simulink model "V2X_Core_Simulink_model"  (R2023b)
settings: Solver=VariableStepAuto  StartTime=0.0  StopTime=210  MaxStep=1e-2  RelTol=1e-3  AbsTol=1e-3
values from neighbouring files (symbols this model uses):
  b = 1.6    [a2024_v2x_matlab_6veh.m]
  mEgo = 1500    [a2024_v2x_matlab_6veh.m]
  Mode = 1    [a2024_v2x_matlab_6veh.m]    (also in v2x_matlab.m; v2x_matlabV2.m; v2x_matlab_6veh.m; v2x_matlab_R.m)
  pilot = (randi(s,[0 1],pilotsPerSym,1)-0.5)*2    [v2x_matlab.m]
  RxPower = [waypoints, ss']    [v2x_matlab.m]    (also in v2x_matlab_6veh.m)
  sampleTime = 0.1    [a2024_v2x_matlab_6veh.m]    (also in v2x_matlab.m; v2x_matlabV2.m; v2x_matlab_6veh.m; v2x_matlab_R.m)
  t_gap = 1.4    [a2024_v2x_matlab_6veh.m]
  waypoints = [egoWP(:,2) egoWP(:,1), zeroforwp]    [a2024_v2x_matlab_6veh.m]    (also in misc.m = data.data.ActorSpecifications(1,1).Waypoints(:,[1,2]); v2x_matlab.m = data.data.ActorSpecifications(1,1).Waypoints(:,[1,2]); v2x_matlabV2.m = [5 -1.6 0; v2x_matlab_R.m = [5 -1.6 0)
  ZeroActors = struct(     'ActorID',0,     'Position', [1000 1000 1000],      'Velocity', [0 0 0],      'Roll', 0,      'Pitch', 0,      'Yaw', 0,      'AngularVelocity', [0 0 0])    [v2x_matlabV2.m]    (also in v2x_matlab_R.m)
undefined symbols (not defined in the file or in its folder): driving, PredictionHorizon, Ts
libraries: commofdm x21, simulink x16, commdigbbndam3 x14, simulink_extras x12, commcnvcod2 x11, commdigbbndpm3 x9, commblkintrlv2 x4, drivingscenarioandsensors x3, mpcadaslib x2, vehdynlibdriver x1, autolibshared x1, commchan3 x1
(part 2 of 4)

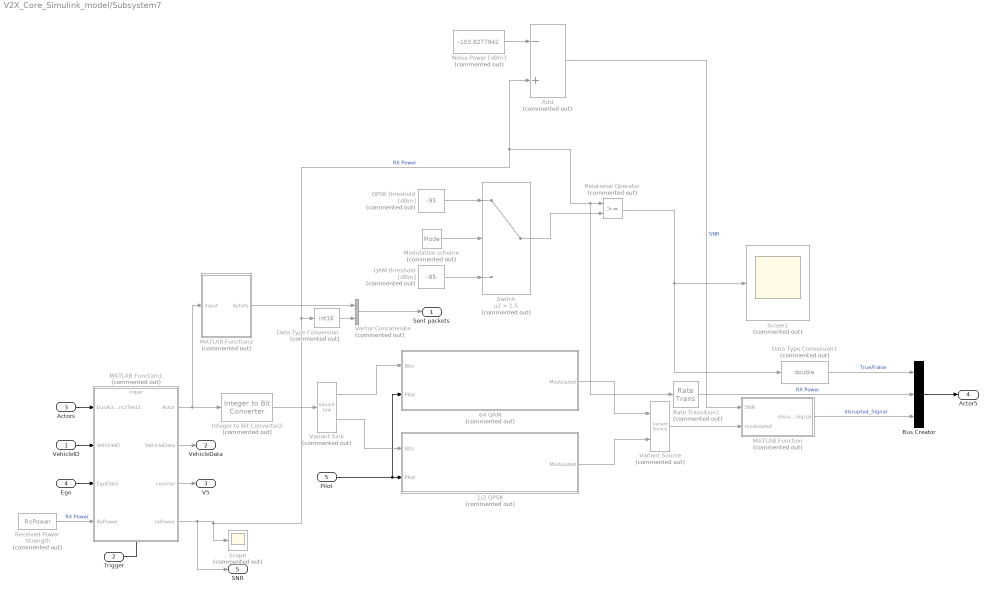
== system V2X_Core_Simulink_model/Subsystem7 ==
  VehicleID : Inport
  Trigger : Inport  Port=2
  Actors : Inport  Port=3
  Ego : Inport  Port=4
  Pilot : Inport  Port=5
  1/2 QPSK : Subsystem  Commented=on  TreatAsAtomicUnit=on
  64 QAM : Subsystem  Commented=on  TreatAsAtomicUnit=on
  Add : Sum  Commented=on  Inputs=-+
  Bus Creator : BusCreator  Inputs=3
  Data Type Conversion : DataTypeConversion  Commented=on  OutDataTypeStr=int16  SaturateOnIntegerOverflow=off  RndMeth=Floor
  Data Type Conversion1 : DataTypeConversion  Commented=on  OutDataTypeStr=double  SaturateOnIntegerOverflow=off  RndMeth=Floor
  Integer to Bit Converter2 : simulink/Logic and Bit Operations/Integer to Bit Converter  Commented=on  nbits=16  signedInputValues=Signed  bitOrder=MSB first  outDtype=boolean
  MATLAB Function : MATLAB Function  Commented=on  TreatAsAtomicUnit=on
  MATLAB Function1 : MATLAB Function  Commented=on  TreatAsAtomicUnit=on
  MATLAB Function2 : MATLAB Function  Commented=on  TreatAsAtomicUnit=on  SystemSampleTime=0.01
  Modulation scheme : Constant  Commented=on  Value=Mode
  Noise Power [dBm] : Constant  Commented=on  Value=-103.8277942
  QAM threshold [dBm] : Constant  Commented=on  Value=-85
  QPSK threshold [dBm] : Constant  Commented=on  Value=-95
  Rate Transition1 : RateTransition  Commented=on  OutPortSampleTime=sampleTime/10
  Received Power Strength : Constant  Commented=on  Value=RxPower
  Relational Operator : RelationalOperator  Commented=on  OutDataTypeStr=boolean  RndMeth=Simplest  InputSameDT=off
  Scope : Scope  Commented=on
  Scope1 : Scope  Commented=on
  Switch : Switch  Commented=on  Criteria=u2 > Threshold  Threshold=1.5  SaturateOnIntegerOverflow=off  InputSameDT=off
  Variant Sink : VariantSink  Commented=on
  Variant Source : VariantSource  Commented=on
  Vector Concatenate : Concatenate  Commented=on
  Sent packets : Outport
  VehicleData : Outport  Port=2
  V5 : Outport  Port=3
  Actor5 : Outport  Port=4
  SNR : Outport  Port=5
  wires:
  MATLAB Function1/1(Actor) -> MATLAB Function2/1(input), Integer to Bit Converter2/1
  Ego/1 -> MATLAB Function1/3(EgoData)
  Actors/1 -> MATLAB Function1/1(busActors3Test1)
  VehicleID/1 -> MATLAB Function1/2(VehicleID)
  MATLAB Function1/2(VehicleData) -> VehicleData/1
  MATLAB Function1/3(counter) -> V5/1
  Trigger/1 -> MATLAB Function1/Trigger
  Integer to Bit Converter2/1 -> Variant Sink/1
  Pilot/1 -> 64 QAM/2(Pilot), 1/2 QPSK/2(Pilot)
  64 QAM/1(Modulated) -> Variant Source/1
  1/2 QPSK/1(Modulated) -> Variant Source/2
  Variant Source/1 -> MATLAB Function/2(modulated)
  Variant Sink/1 -> 64 QAM/1(Bits)
  Variant Sink/2 -> 1/2 QPSK/1(Bits)
  Noise Power [dBm]/1 -> Add/1
  QPSK threshold [dBm]/1 -> Switch/1
  QAM threshold [dBm]/1 -> Switch/3
  Modulation scheme/1 -> Switch/2
  Add/1 -> MATLAB Function/1(SNR)  "SNR"
  Switch/1 -> Relational Operator/2
  Relational Operator/1 -> Data Type Conversion1/1, Scope1/1
  MATLAB Function1/4(rxPower) -> Data Type Conversion/1, Rate Transition1/1, Relational Operator/1, Add/2, Scope/1, SNR/1  "RX Power"
  Received Power Strength/1 -> MATLAB Function1/4(RxPower)  "RX Power"
  Bus Creator/1 -> Actor5/1
  MATLAB Function2/1(Actors) -> Vector Concatenate/1
  Vector Concatenate/1 -> Sent packets/1
  MATLAB Function/1(disrupted_Signal) -> Bus Creator/3  "disrupted_Signal"
  Data Type Conversion/1 -> Vector Concatenate/2
  Data Type Conversion1/1 -> Bus Creator/1  "True/False"
  Rate Transition1/1 -> Bus Creator/2  "RX Power"

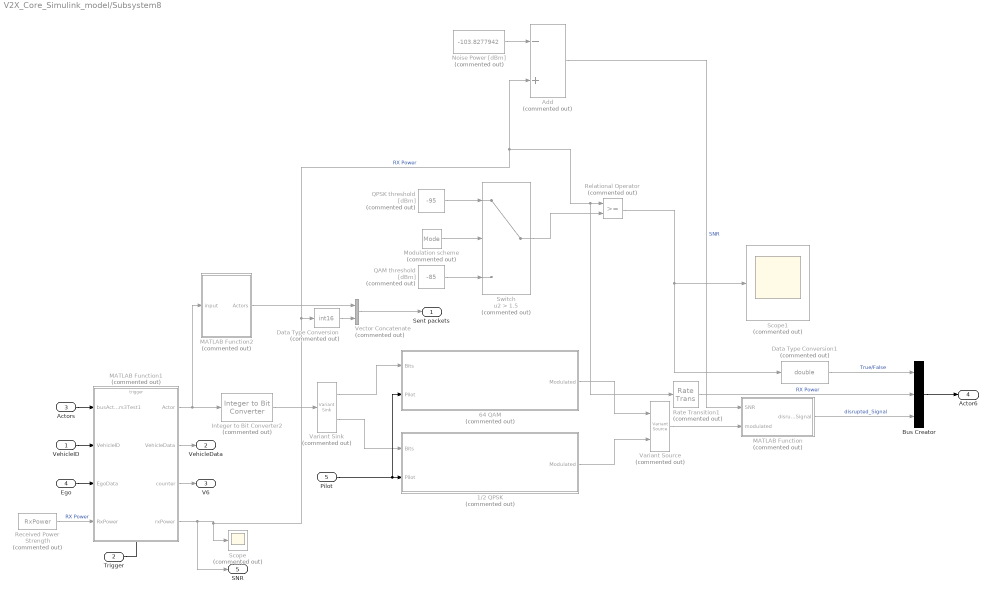
== system V2X_Core_Simulink_model/Subsystem8 ==
  VehicleID : Inport
  Trigger : Inport  Port=2
  Actors : Inport  Port=3
  Ego : Inport  Port=4
  Pilot : Inport  Port=5
  1/2 QPSK : Subsystem  Commented=on  TreatAsAtomicUnit=on
  64 QAM : Subsystem  Commented=on  TreatAsAtomicUnit=on
  Add : Sum  Commented=on  Inputs=-+
  Bus Creator : BusCreator  Inputs=3
  Data Type Conversion : DataTypeConversion  Commented=on  OutDataTypeStr=int16  SaturateOnIntegerOverflow=off  RndMeth=Floor
  Data Type Conversion1 : DataTypeConversion  Commented=on  OutDataTypeStr=double  SaturateOnIntegerOverflow=off  RndMeth=Floor
  Integer to Bit Converter2 : simulink/Logic and Bit Operations/Integer to Bit Converter  Commented=on  nbits=16  signedInputValues=Signed  bitOrder=MSB first  outDtype=boolean
  MATLAB Function : MATLAB Function  Commented=on  TreatAsAtomicUnit=on
  MATLAB Function1 : MATLAB Function  Commented=on  TreatAsAtomicUnit=on
  MATLAB Function2 : MATLAB Function  Commented=on  TreatAsAtomicUnit=on  SystemSampleTime=0.01
  Modulation scheme : Constant  Commented=on  Value=Mode
  Noise Power [dBm] : Constant  Commented=on  Value=-103.8277942
  QAM threshold [dBm] : Constant  Commented=on  Value=-85
  QPSK threshold [dBm] : Constant  Commented=on  Value=-95
  Rate Transition1 : RateTransition  Commented=on  OutPortSampleTime=sampleTime/10
  Received Power Strength : Constant  Commented=on  Value=RxPower
  Relational Operator : RelationalOperator  Commented=on  OutDataTypeStr=boolean  RndMeth=Simplest  InputSameDT=off
  Scope : Scope  Commented=on
  Scope1 : Scope  Commented=on
  Switch : Switch  Commented=on  Criteria=u2 > Threshold  Threshold=1.5  SaturateOnIntegerOverflow=off  InputSameDT=off
  Variant Sink : VariantSink  Commented=on
  Variant Source : VariantSource  Commented=on
  Vector Concatenate : Concatenate  Commented=on
  Sent packets : Outport
  VehicleData : Outport  Port=2
  V6 : Outport  Port=3
  Actor6 : Outport  Port=4
  SNR : Outport  Port=5
  wires:
  Rate Transition1/1 -> Bus Creator/2  "RX Power"
  Data Type Conversion1/1 -> Bus Creator/1  "True/False"
  Data Type Conversion/1 -> Vector Concatenate/2
  MATLAB Function/1(disrupted_Signal) -> Bus Creator/3  "disrupted_Signal"
  Vector Concatenate/1 -> Sent packets/1
  MATLAB Function2/1(Actors) -> Vector Concatenate/1
  Bus Creator/1 -> Actor6/1
  Received Power Strength/1 -> MATLAB Function1/4(RxPower)  "RX Power"
  MATLAB Function1/4(rxPower) -> SNR/1, Scope/1, Add/2, Relational Operator/1, Rate Transition1/1, Data Type Conversion/1  "RX Power"
  Relational Operator/1 -> Scope1/1, Data Type Conversion1/1
  Switch/1 -> Relational Operator/2
  Add/1 -> MATLAB Function/1(SNR)  "SNR"
  Modulation scheme/1 -> Switch/2
  QAM threshold [dBm]/1 -> Switch/3
  QPSK threshold [dBm]/1 -> Switch/1
  Noise Power [dBm]/1 -> Add/1
  Variant Sink/2 -> 1/2 QPSK/1(Bits)
  Variant Sink/1 -> 64 QAM/1(Bits)
  Variant Source/1 -> MATLAB Function/2(modulated)
  1/2 QPSK/1(Modulated) -> Variant Source/2
  64 QAM/1(Modulated) -> Variant Source/1
  Pilot/1 -> 1/2 QPSK/2(Pilot), 64 QAM/2(Pilot)
  Integer to Bit Converter2/1 -> Variant Sink/1
  Trigger/1 -> MATLAB Function1/Trigger
  MATLAB Function1/3(counter) -> V6/1
  MATLAB Function1/2(VehicleData) -> VehicleData/1
  VehicleID/1 -> MATLAB Function1/2(VehicleID)
  Actors/1 -> MATLAB Function1/1(busActors3Test1)
  Ego/1 -> MATLAB Function1/3(EgoData)
  MATLAB Function1/1(Actor) -> Integer to Bit Converter2/1, MATLAB Function2/1(input)

== system V2X_Core_Simulink_model/Vehicle 2 ==
  trigger : Inport
  VehicleID : Inport  Port=2
  Pilot : Inport  Port=3
  busActors3Test1 : Inport  Port=4
  Constant2 : Constant  Value=[zeros(19,1)']  SampleTime=-1
  Entity Multicast1 : EntityMulticast  InputPortMessageModes=m
  Integer to Bit Converter1 : simulink/Logic and Bit Operations/Integer to Bit Converter  nbits=16  signedInputValues=Signed  bitOrder=MSB first  outDtype=boolean
  MATLAB Function1 : MATLAB Function  TreatAsAtomicUnit=on
  OFDM Modulator1 : commofdm/OFDM Modulator  StatePerturbationForJacobian=1.0e-05  FFTLength=64  NumGuardBandCarriers=[0;0]  InsertDCNull=on  PilotInputPort=on  PilotCarrierIndices=[12; 26; 40; 54]  CyclicPrefixLength=32  Windowing=off  WindowLength=16  OversamplingFactor=3  NumSymbols=1  NumTransmitAntennas=1  SimulateUsing=Interpreted execution
  Rectangular QAM Modulator Baseband1 : commdigbbndam3/Rectangular QAM Modulator Baseband  M=2^6  InType=Bit  Enc=Binary  Mapping=[0:15]  PowType=Average Power  MinDist=2  AvgPow=P_Signal  PeakPow=1  Ph=0  outDtype=double  outWordLen=16  outUDDataType=sfix(16)  outFracLenMode=Best precision  outFracLen=15  outDataTypeStr=double  outLastDataTypeStr=double
      settings: LibrarySourceBlock=|
      | commhdldigbbndam/Rectangular QAM
      | Modulator
      | Baseband
  Send1 : Send  OutputPortMessageModes=m
  Vector Concatenate1 : Concatenate
  wires:
  busActors3Test1/1 -> MATLAB Function1/1(busActors3Test1)
  Rectangular QAM Modulator Baseband1/1 -> Vector Concatenate1/1
  Constant2/1 -> Vector Concatenate1/2
  Send1/1 -> Entity Multicast1/1
  Integer to Bit Converter1/1 -> Rectangular QAM Modulator Baseband1/1
  Vector Concatenate1/1 -> OFDM Modulator1/1  "After QAM Mod"
  OFDM Modulator1/1 -> Send1/1  "OFDM modulated"
  MATLAB Function1/1(intVector) -> Integer to Bit Converter1/1
  trigger/1 -> MATLAB Function1/Trigger
  VehicleID/1 -> MATLAB Function1/2(VehicleID)
  Pilot/1 -> OFDM Modulator1/2

== system V2X_Core_Simulink_model/Vehicle 3 ==
  trigger : Inport
  busActors3Test1 : Inport  Port=2
  Pilot : Inport  Port=3
  VehicleID : Inport  Port=4
  Constant3 : Constant  Value=[zeros(19,1)']  SampleTime=-1
  Entity Multicast2 : EntityMulticast  InputPortMessageModes=m
  Integer to Bit Converter3 : simulink/Logic and Bit Operations/Integer to Bit Converter  nbits=16  signedInputValues=Signed  bitOrder=MSB first  outDtype=boolean
  MATLAB Function2 : MATLAB Function  TreatAsAtomicUnit=on
  OFDM Modulator2 : commofdm/OFDM Modulator  StatePerturbationForJacobian=1.0e-05  FFTLength=64  NumGuardBandCarriers=[0;0]  InsertDCNull=on  PilotInputPort=on  PilotCarrierIndices=[12; 26; 40; 54]  CyclicPrefixLength=32  Windowing=off  WindowLength=16  OversamplingFactor=3  NumSymbols=1  NumTransmitAntennas=1  SimulateUsing=Interpreted execution
  Rectangular QAM Modulator Baseband3 : commdigbbndam3/Rectangular QAM Modulator Baseband  M=2^6  InType=Bit  Enc=Binary  Mapping=[0:15]  PowType=Average Power  MinDist=2  AvgPow=P_Signal  PeakPow=1  Ph=0  outDtype=double  outWordLen=16  outUDDataType=sfix(16)  outFracLenMode=Best precision  outFracLen=15  outDataTypeStr=double  outLastDataTypeStr=double
      settings: LibrarySourceBlock=|
      | commhdldigbbndam/Rectangular QAM
      | Modulator
      | Baseband
  Send2 : Send  OutputPortMessageModes=m
  Vector Concatenate2 : Concatenate
  wires:
  MATLAB Function2/1(intVector) -> Integer to Bit Converter3/1
  OFDM Modulator2/1 -> Send2/1  "OFDM modulated"
  busActors3Test1/1 -> MATLAB Function2/1(busActors3Test1)
  Vector Concatenate2/1 -> OFDM Modulator2/1  "After QAM Mod"
  Send2/1 -> Entity Multicast2/1
  Integer to Bit Converter3/1 -> Rectangular QAM Modulator Baseband3/1
  Rectangular QAM Modulator Baseband3/1 -> Vector Concatenate2/1
  Pilot/1 -> OFDM Modulator2/2
  Constant3/1 -> Vector Concatenate2/2
  VehicleID/1 -> MATLAB Function2/2(VehicleID)
  trigger/1 -> MATLAB Function2/Trigger

== system V2X_Core_Simulink_model/ACC/Lane Keeping Assist ==
  Longitudinal velocity of ego : Inport
  Enable : Inport  Port=2
  Lane Assist Offset : Inport  Port=3
  lane boundaries Bus : Inport  Port=4
  Driver Steer : Inport  Port=5
  Abs : Abs  SaturateOnIntegerOverflow=off
  Estimate lane center : Subsystem
  Lane Keeping Assist System : mpcadaslib/Lane Keeping Assist System  ModelType=Use vehicle parameters  VehicleMass=mEgo  VehicleYawInertia=2875  LengthToFront=a  LengthToRear=b  FrontTireStiffness=Cy_f  RearTireStiffness=Cy_r  EgoModelMatrixA=[-4.4021 ,-12.4603;1.3913,-5.1868]  EgoModelMatrixB=[24.1270;15.8609]  EgoModelMatrixC=[1,0;0,1]  InitialLongVel=16  TransportLag=0  MinSteering=-0.5  umin_ext=off  MaxSteering=0.5  umax_ext=off  Ts=0.1  PredictionHorizon=5  ControllerBehavior=0.100  suboptimal=off  maxiter=10  datatypeopt=double  optmode=off  trackmode=off
      link override Longitudinal velocity must be positive: stopWhenAssertionFail=on
      settings: LibrarySourceBlock=mpclib/Automated Driving/Lane Keeping Assist System
  Pack to Custom Sensor Data Format : Subsystem
  Subsystem : Subsystem
  Subsystem2 : Subsystem
  Vision Detection Generator : drivingscenarioandsensors/Vision Detection Generator  SensorIndex=1  DetectorOutput=Lanes only  UpdateInterval=0.1  LaneUpdateInterval=0.1  SensorLocation=[ 1.9, 0 ]  Height=1.1  Yaw=0  Pitch=1  Roll=0  BusNameSource=Auto  BusName=BusObjectDetections  BusName2Source=Auto  BusName2=BusLaneDetections  MaxNumDetectionsSource=Property  MaxNumDetections=50  MaxNumLanesSource=Property  MaxNumLanes=30  DetectionCoordinates=Ego Cartesian  SimulateUsing=Interpreted execution  MaxRange=10  BoundingBoxAccuracy=5  ProcessNoiseIntensity=5  MaxSpeed=100  MaxAllowedOcclusion=0.5  MinObjectImageSize=[ 15, 15 ]  DetectionProbability=0.9  FalsePositivesPerImage=0.1  MinLaneImageSize=[ 20, 3 ]  LaneBoundaryAccuracy=3  HasNoise=on  InitialSeedSource=Repeatable  InitialSeed=0  UsedSeed=driving.internal.SimulinkUtilities.seedManager(gcb)  ActorProfilesSource=From Scenario Reader block  ActorProfilesParameters=driving.internal.ActorProfilesParameters  ActorProfilesExpression=struct( 'ClassID', 0, 'Length', 4.7, 'Width', 1.8, 'Height', 1.4, 'OriginOffset', [ -1.35, 0, 0 ] )  Intrinsics=driving.internal.cameraIntrinsics('FocalLength',[1, 1 ])
  Status : Outport
  SteeringAngle in rad : Outport  Port=2
  wires:
  Subsystem/1(Departure Detected) -> Subsystem2/2(Set)
  Estimate lane center/2(Lateral Offset) -> Lane Keeping Assist System/3
  Enable/1 -> Subsystem2/1(Enable)
  Pack to Custom Sensor Data Format/1(lanes) -> Subsystem/2(Lane Sensor data), Estimate lane center/2(Lane Boundaries)
  Estimate lane center/1(Previewed Curvature) -> Lane Keeping Assist System/1
  Estimate lane center/3(Heading Angle) -> Lane Keeping Assist System/4
  lane boundaries Bus/1 -> Vision Detection Generator/1
  Vision Detection Generator/1 -> Pack to Custom Sensor Data Format/1(lane Detections)
  Lane Assist Offset/1 -> Subsystem/1(Lane Assist Offset)
  Driver Steer/1 -> Subsystem2/4(Driver Steer)
  Subsystem2/1(Status) -> Status/1
  Longitudinal velocity of ego/1 -> Abs/1, Estimate lane center/1(Longitudinal velocity of ego)
  Abs/1 -> Lane Keeping Assist System/2
  Subsystem2/2(SteeringAngle in rad) -> SteeringAngle in rad/1
  Lane Keeping Assist System/1 -> Subsystem2/3(Assisted Steer)  "Assisted Steer"

== system V2X_Core_Simulink_model/Calculate PDR/PDR V1 ==
  Sent packet : Inport
  Received packets : Inport  Port=2
  Vehicle ID : Inport  Port=3
  Add : Sum  Commented=on  Inputs=-+
  Bus Selector3 : BusSelector  Commented=on  OutputSignals=ActorID,Position,Velocity,Roll,Pitch,Yaw,AngularVelocity
  Constant : Constant  Commented=on
  Data Type Conversion1 : DataTypeConversion  Commented=on  OutDataTypeStr=double  SaturateOnIntegerOverflow=off  RndMeth=Floor
  MATLAB Function : MATLAB Function  TreatAsAtomicUnit=on
  MATLAB Function1 : MATLAB Function  TreatAsAtomicUnit=on
  MATLAB Function2 : MATLAB Function  TreatAsAtomicUnit=on
  MATLAB Function6 : MATLAB Function  Commented=on  TreatAsAtomicUnit=on
  Matrix Concatenate : Concatenate  Mode=Multidimensional array  ConcatenateDimension=2
  Round : Rounding  Commented=on  Operator=round
  Selector : Selector  Commented=through  IndexOptions=Starting index (dialog)  Indices=3  OutputSizes=13
  Transpose : Math  Commented=on  Operator=transpose
  Vector Concatenate1 : Concatenate  Commented=on  NumInputs=7
  PDR1 : Outport
  Vectors output : Outport  Port=2
  wires:
  MATLAB Function2/1(y) -> Selector/1
  Received packets/1 -> MATLAB Function2/2(u)
  MATLAB Function1/1(y) -> Matrix Concatenate/1, MATLAB Function/1(Tx)
  MATLAB Function/1(PDR) -> PDR1/1
  Matrix Concatenate/1 -> Vectors output/1
  Selector/1 -> MATLAB Function/2(Rx), Matrix Concatenate/2
  Vehicle ID/1 -> MATLAB Function1/2(Vehicle_ID), MATLAB Function2/1(Vehicle_ID)
  ? -> MATLAB Function6/2(vehicleID)
  Bus Selector3/6 -> Vector Concatenate1/6  "<Yaw>"
  Bus Selector3/4 -> Vector Concatenate1/4  "<Roll>"
  Constant/1 -> Add/1
  Bus Selector3/7 -> Vector Concatenate1/7  "<AngularVelocity>"
  Vector Concatenate1/1 -> Transpose/1
  Add/1 -> Vector Concatenate1/1
  MATLAB Function6/1(y) -> Bus Selector3/1
  Bus Selector3/3 -> Vector Concatenate1/3  "<Velocity>"
  Bus Selector3/2 -> Vector Concatenate1/2  "<Position>"
  ? -> MATLAB Function6/1(u)
  Bus Selector3/5 -> Vector Concatenate1/5  "<Pitch>"
  Bus Selector3/1 -> Add/2  "<ActorID>"
  Transpose/1 -> Round/1
  Round/1 -> Data Type Conversion1/1
  Sent packet/1 -> MATLAB Function1/1(u)

== system V2X_Core_Simulink_model/Calculate PDR/PDR V2 ==
  Sent packet : Inport
  Received packets : Inport  Port=2
  Vehicle ID : Inport  Port=3
  Add : Sum  Commented=on  Inputs=-+
  Bus Selector3 : BusSelector  Commented=on  OutputSignals=ActorID,Position,Velocity,Roll,Pitch,Yaw,AngularVelocity
  Constant : Constant  Commented=on
  Data Type Conversion1 : DataTypeConversion  Commented=on  OutDataTypeStr=double  SaturateOnIntegerOverflow=off  RndMeth=Floor
  MATLAB Function : MATLAB Function  TreatAsAtomicUnit=on
  MATLAB Function1 : MATLAB Function  TreatAsAtomicUnit=on
  MATLAB Function2 : MATLAB Function  TreatAsAtomicUnit=on
  MATLAB Function6 : MATLAB Function  Commented=on  TreatAsAtomicUnit=on
  Matrix Concatenate : Concatenate  Mode=Multidimensional array  ConcatenateDimension=2
  Round : Rounding  Commented=on  Operator=round
  Selector : Selector  Commented=through  IndexOptions=Starting index (dialog)  Indices=3  OutputSizes=13
  Transpose : Math  Commented=on  Operator=transpose
  Vector Concatenate1 : Concatenate  Commented=on  NumInputs=7
  PDR1 : Outport
  Vectors output : Outport  Port=2
  wires:
  Sent packet/1 -> MATLAB Function1/1(u)
  Round/1 -> Data Type Conversion1/1
  Transpose/1 -> Round/1
  Bus Selector3/1 -> Add/2  "<ActorID>"
  Bus Selector3/5 -> Vector Concatenate1/5  "<Pitch>"
  ? -> MATLAB Function6/1(u)
  Bus Selector3/2 -> Vector Concatenate1/2  "<Position>"
  Bus Selector3/3 -> Vector Concatenate1/3  "<Velocity>"
  MATLAB Function6/1(y) -> Bus Selector3/1
  Add/1 -> Vector Concatenate1/1
  Vector Concatenate1/1 -> Transpose/1
  Bus Selector3/7 -> Vector Concatenate1/7  "<AngularVelocity>"
  Constant/1 -> Add/1
  Bus Selector3/4 -> Vector Concatenate1/4  "<Roll>"
  Bus Selector3/6 -> Vector Concatenate1/6  "<Yaw>"
  ? -> MATLAB Function6/2(vehicleID)
  Vehicle ID/1 -> MATLAB Function2/1(Vehicle_ID), MATLAB Function1/2(Vehicle_ID)
  Selector/1 -> Matrix Concatenate/2, MATLAB Function/2(Rx)
  Matrix Concatenate/1 -> Vectors output/1
  MATLAB Function/1(PDR) -> PDR1/1
  MATLAB Function1/1(y) -> MATLAB Function/1(Tx), Matrix Concatenate/1
  Received packets/1 -> MATLAB Function2/2(u)
  MATLAB Function2/1(y) -> Selector/1

== system V2X_Core_Simulink_model/Calculate PDR/PDR V3 ==
  Sent packet : Inport
  Received packets : Inport  Port=2
  Vehicle ID : Inport  Port=3
  Add : Sum  Commented=on  Inputs=-+
  Bus Selector3 : BusSelector  Commented=on  OutputSignals=ActorID,Position,Velocity,Roll,Pitch,Yaw,AngularVelocity
  Constant : Constant  Commented=on
  Data Type Conversion1 : DataTypeConversion  Commented=on  OutDataTypeStr=double  SaturateOnIntegerOverflow=off  RndMeth=Floor
  MATLAB Function : MATLAB Function  TreatAsAtomicUnit=on
  MATLAB Function1 : MATLAB Function  TreatAsAtomicUnit=on
  MATLAB Function2 : MATLAB Function  TreatAsAtomicUnit=on
  MATLAB Function6 : MATLAB Function  Commented=on  TreatAsAtomicUnit=on
  Matrix Concatenate : Concatenate  Mode=Multidimensional array  ConcatenateDimension=2
  Round : Rounding  Commented=on  Operator=round
  Selector : Selector  Commented=through  IndexOptions=Starting index (dialog)  Indices=3  OutputSizes=13
  Transpose : Math  Commented=on  Operator=transpose
  Vector Concatenate1 : Concatenate  Commented=on  NumInputs=7
  PDR1 : Outport
  Vectors output : Outport  Port=2
  wires:
  MATLAB Function2/1(y) -> Selector/1
  Received packets/1 -> MATLAB Function2/2(u)
  MATLAB Function1/1(y) -> Matrix Concatenate/1, MATLAB Function/1(Tx)
  MATLAB Function/1(PDR) -> PDR1/1
  Matrix Concatenate/1 -> Vectors output/1
  Selector/1 -> MATLAB Function/2(Rx), Matrix Concatenate/2
  Vehicle ID/1 -> MATLAB Function1/2(Vehicle_ID), MATLAB Function2/1(Vehicle_ID)
  ? -> MATLAB Function6/2(vehicleID)
  Bus Selector3/6 -> Vector Concatenate1/6  "<Yaw>"
  Bus Selector3/4 -> Vector Concatenate1/4  "<Roll>"
  Constant/1 -> Add/1
  Bus Selector3/7 -> Vector Concatenate1/7  "<AngularVelocity>"
  Vector Concatenate1/1 -> Transpose/1
  Add/1 -> Vector Concatenate1/1
  MATLAB Function6/1(y) -> Bus Selector3/1
  Bus Selector3/3 -> Vector Concatenate1/3  "<Velocity>"
  Bus Selector3/2 -> Vector Concatenate1/2  "<Position>"
  ? -> MATLAB Function6/1(u)
  Bus Selector3/5 -> Vector Concatenate1/5  "<Pitch>"
  Bus Selector3/1 -> Add/2  "<ActorID>"
  Transpose/1 -> Round/1
  Round/1 -> Data Type Conversion1/1
  Sent packet/1 -> MATLAB Function1/1(u)

== system V2X_Core_Simulink_model/Calculate PDR/PDR V4 ==
  Sent packet : Inport
  Received packets : Inport  Port=2
  Vehicle ID : Inport  Port=3
  Add : Sum  Commented=on  Inputs=-+
  Bus Selector3 : BusSelector  Commented=on  OutputSignals=ActorID,Position,Velocity,Roll,Pitch,Yaw,AngularVelocity
  Constant : Constant  Commented=on
  Data Type Conversion1 : DataTypeConversion  Commented=on  OutDataTypeStr=double  SaturateOnIntegerOverflow=off  RndMeth=Floor
  MATLAB Function : MATLAB Function  TreatAsAtomicUnit=on
  MATLAB Function1 : MATLAB Function  TreatAsAtomicUnit=on
  MATLAB Function2 : MATLAB Function  TreatAsAtomicUnit=on
  MATLAB Function6 : MATLAB Function  Commented=on  TreatAsAtomicUnit=on
  Matrix Concatenate : Concatenate  Mode=Multidimensional array  ConcatenateDimension=2
  Round : Rounding  Commented=on  Operator=round
  Selector : Selector  Commented=through  IndexOptions=Starting index (dialog)  Indices=3  OutputSizes=13
  Transpose : Math  Commented=on  Operator=transpose
  Vector Concatenate1 : Concatenate  Commented=on  NumInputs=7
  PDR1 : Outport
  Vectors output : Outport  Port=2
  wires:
  Sent packet/1 -> MATLAB Function1/1(u)
  Round/1 -> Data Type Conversion1/1
  Transpose/1 -> Round/1
  Bus Selector3/1 -> Add/2  "<ActorID>"
  Bus Selector3/5 -> Vector Concatenate1/5  "<Pitch>"
  ? -> MATLAB Function6/1(u)
  Bus Selector3/2 -> Vector Concatenate1/2  "<Position>"
  Bus Selector3/3 -> Vector Concatenate1/3  "<Velocity>"
  MATLAB Function6/1(y) -> Bus Selector3/1
  Add/1 -> Vector Concatenate1/1
  Vector Concatenate1/1 -> Transpose/1
  Bus Selector3/7 -> Vector Concatenate1/7  "<AngularVelocity>"
  Constant/1 -> Add/1
  Bus Selector3/4 -> Vector Concatenate1/4  "<Roll>"
  Bus Selector3/6 -> Vector Concatenate1/6  "<Yaw>"
  ? -> MATLAB Function6/2(vehicleID)
  Vehicle ID/1 -> MATLAB Function2/1(Vehicle_ID), MATLAB Function1/2(Vehicle_ID)
  Selector/1 -> Matrix Concatenate/2, MATLAB Function/2(Rx)
  Matrix Concatenate/1 -> Vectors output/1
  MATLAB Function/1(PDR) -> PDR1/1
  MATLAB Function1/1(y) -> MATLAB Function/1(Tx), Matrix Concatenate/1
  Received packets/1 -> MATLAB Function2/2(u)
  MATLAB Function2/1(y) -> Selector/1

== system V2X_Core_Simulink_model/Calculate PDR/PDR V5 ==
  Sent packet : Inport
  Received packets : Inport  Port=2
  Vehicle ID : Inport  Port=3
  Add : Sum  Commented=on  Inputs=-+
  Bus Selector3 : BusSelector  Commented=on  OutputSignals=ActorID,Position,Velocity,Roll,Pitch,Yaw,AngularVelocity
  Constant : Constant  Commented=on
  Data Type Conversion1 : DataTypeConversion  Commented=on  OutDataTypeStr=double  SaturateOnIntegerOverflow=off  RndMeth=Floor
  MATLAB Function : MATLAB Function  TreatAsAtomicUnit=on
  MATLAB Function1 : MATLAB Function  TreatAsAtomicUnit=on
  MATLAB Function2 : MATLAB Function  TreatAsAtomicUnit=on
  MATLAB Function6 : MATLAB Function  Commented=on  TreatAsAtomicUnit=on
  Matrix Concatenate : Concatenate  Mode=Multidimensional array  ConcatenateDimension=2
  Round : Rounding  Commented=on  Operator=round
  Selector : Selector  Commented=through  IndexOptions=Starting index (dialog)  Indices=3  OutputSizes=13
  Transpose : Math  Commented=on  Operator=transpose
  Vector Concatenate1 : Concatenate  Commented=on  NumInputs=7
  PDR1 : Outport
  Vectors output : Outport  Port=2
  wires:
  MATLAB Function2/1(y) -> Selector/1
  Received packets/1 -> MATLAB Function2/2(u)
  MATLAB Function1/1(y) -> Matrix Concatenate/1, MATLAB Function/1(Tx)
  MATLAB Function/1(PDR) -> PDR1/1
  Matrix Concatenate/1 -> Vectors output/1
  Selector/1 -> MATLAB Function/2(Rx), Matrix Concatenate/2
  Vehicle ID/1 -> MATLAB Function1/2(Vehicle_ID), MATLAB Function2/1(Vehicle_ID)
  ? -> MATLAB Function6/2(vehicleID)
  Bus Selector3/6 -> Vector Concatenate1/6  "<Yaw>"
  Bus Selector3/4 -> Vector Concatenate1/4  "<Roll>"
  Constant/1 -> Add/1
  Bus Selector3/7 -> Vector Concatenate1/7  "<AngularVelocity>"
  Vector Concatenate1/1 -> Transpose/1
  Add/1 -> Vector Concatenate1/1
  MATLAB Function6/1(y) -> Bus Selector3/1
  Bus Selector3/3 -> Vector Concatenate1/3  "<Velocity>"
  Bus Selector3/2 -> Vector Concatenate1/2  "<Position>"
  ? -> MATLAB Function6/1(u)
  Bus Selector3/5 -> Vector Concatenate1/5  "<Pitch>"
  Bus Selector3/1 -> Add/2  "<ActorID>"
  Transpose/1 -> Round/1
  Round/1 -> Data Type Conversion1/1
  Sent packet/1 -> MATLAB Function1/1(u)

== system V2X_Core_Simulink_model/Calculate PDR/PDR V6 ==
  Sent packet : Inport
  Received packets : Inport  Port=2
  Vehicle ID : Inport  Port=3
  Add : Sum  Commented=on  Inputs=-+
  Bus Selector3 : BusSelector  Commented=on  OutputSignals=ActorID,Position,Velocity,Roll,Pitch,Yaw,AngularVelocity
  Constant : Constant  Commented=on
  Data Type Conversion1 : DataTypeConversion  Commented=on  OutDataTypeStr=double  SaturateOnIntegerOverflow=off  RndMeth=Floor
  MATLAB Function : MATLAB Function  TreatAsAtomicUnit=on
  MATLAB Function1 : MATLAB Function  TreatAsAtomicUnit=on
  MATLAB Function2 : MATLAB Function  TreatAsAtomicUnit=on
  MATLAB Function6 : MATLAB Function  Commented=on  TreatAsAtomicUnit=on
  Matrix Concatenate : Concatenate  Mode=Multidimensional array  ConcatenateDimension=2
  Round : Rounding  Commented=on  Operator=round
  Selector : Selector  Commented=through  IndexOptions=Starting index (dialog)  Indices=3  OutputSizes=13
  Transpose : Math  Commented=on  Operator=transpose
  Vector Concatenate1 : Concatenate  Commented=on  NumInputs=7
  PDR1 : Outport
  Vectors output : Outport  Port=2
  wires:
  Sent packet/1 -> MATLAB Function1/1(u)
  Round/1 -> Data Type Conversion1/1
  Transpose/1 -> Round/1
  Bus Selector3/1 -> Add/2  "<ActorID>"
  Bus Selector3/5 -> Vector Concatenate1/5  "<Pitch>"
  ? -> MATLAB Function6/1(u)
  Bus Selector3/2 -> Vector Concatenate1/2  "<Position>"
  Bus Selector3/3 -> Vector Concatenate1/3  "<Velocity>"
  MATLAB Function6/1(y) -> Bus Selector3/1
  Add/1 -> Vector Concatenate1/1
  Vector Concatenate1/1 -> Transpose/1
  Bus Selector3/7 -> Vector Concatenate1/7  "<AngularVelocity>"
  Constant/1 -> Add/1
  Bus Selector3/4 -> Vector Concatenate1/4  "<Roll>"
  Bus Selector3/6 -> Vector Concatenate1/6  "<Yaw>"
  ? -> MATLAB Function6/2(vehicleID)
  Vehicle ID/1 -> MATLAB Function2/1(Vehicle_ID), MATLAB Function1/2(Vehicle_ID)
  Selector/1 -> Matrix Concatenate/2, MATLAB Function/2(Rx)
  Matrix Concatenate/1 -> Vectors output/1
  MATLAB Function/1(PDR) -> PDR1/1
  MATLAB Function1/1(y) -> MATLAB Function/1(Tx), Matrix Concatenate/1
  Received packets/1 -> MATLAB Function2/2(u)
  MATLAB Function2/1(y) -> Selector/1

== system V2X_Core_Simulink_model/Queue/Switch Case Action Subsystem ==
  Actor1 : Inport
  Action Port : ActionPort  ActionPortLabel=case [ 0 ]:
  Out1 : Outport
  wires:
  Actor1/1 -> Out1/1

== system V2X_Core_Simulink_model/Queue/Switch Case Action Subsystem1 ==
  Actor1 : Inport
  Action Port : ActionPort  ActionPortLabel=case [ 1 ]:
  Out1 : Outport
  wires:
  Actor1/1 -> Out1/1

== system V2X_Core_Simulink_model/Queue/Switch Case Action Subsystem2 ==
  Actor1 : Inport
  Action Port : ActionPort  ActionPortLabel=case [ 2 ]:
  Out1 : Outport
  wires:
  Actor1/1 -> Out1/1

== system V2X_Core_Simulink_model/Queue/Switch Case Action Subsystem3 ==
  Actor1 : Inport
  Action Port : ActionPort  ActionPortLabel=case [ 3 ]:
  Out1 : Outport
  wires:
  Actor1/1 -> Out1/1

== system V2X_Core_Simulink_model/Queue/Switch Case Action Subsystem4 ==
  Actor1 : Inport
  Action Port : ActionPort  ActionPortLabel=case [ 4 ]:
  Out1 : Outport
  wires:
  Actor1/1 -> Out1/1

== system V2X_Core_Simulink_model/Queue/Switch Case Action Subsystem5 ==
  Actor1 : Inport
  Action Port : ActionPort  ActionPortLabel=case [ 5 ]:
  Out1 : Outport
  wires:
  Actor1/1 -> Out1/1

== system V2X_Core_Simulink_model/Subsystem/1//2 64 QAM ==
  Bits : Inport
  Pilot : Inport  Port=2
  Constant2 : Constant  Value=[zeros(887,1)]  VectorParams1D=off  SampleTime=-1
  Convolutional Encoder : commcnvcod2/Convolutional Encoder  trellis=poly2trellis(7, [171 133])  opMode=Truncated (reset every frame)  DelayedResetAction=on  hasIniStPort=off  hasFinStPort=off  usePuncVector=off  punctureVector=[1;1;0;1;1;0;1;1;0;1;0;1;1;0;1;1;0;1]  reset=Unused parameter value
      settings: LibrarySourceBlock=|
      | commhdlcnvcod/Convolutional
      | Encoder
  Display : Display
  OFDM Modulator1 : commofdm/OFDM Modulator  StatePerturbationForJacobian=1.0e-05  FFTLength=1024  NumGuardBandCarriers=[0;0]  InsertDCNull=on  PilotInputPort=on  PilotCarrierIndices=pilotInd  CyclicPrefixLength=512  Windowing=off  WindowLength=16  OversamplingFactor=1  NumSymbols=1  NumTransmitAntennas=1  SimulateUsing=Interpreted execution
  Rectangular QAM Modulator Baseband2 : commdigbbndam3/Rectangular QAM Modulator Baseband  M=2^6  InType=Bit  Enc=Gray  Mapping=[0:15]  PowType=Average Power  MinDist=2  AvgPow=42  PeakPow=1  Ph=0  outDtype=double  outWordLen=16  outUDDataType=sfix(16)  outFracLenMode=Best precision  outFracLen=15  outDataTypeStr=double  outLastDataTypeStr=double
      settings: LibrarySourceBlock=|
      | commhdldigbbndam/Rectangular QAM
      | Modulator
      | Baseband
  Vector Concatenate : Concatenate
  Modulated : Outport
  wires:
  Bits/1 -> Convolutional Encoder/1  "Raw"
  Vector Concatenate/1 -> OFDM Modulator1/1  "After QAM Mod"
  Constant2/1 -> Vector Concatenate/2
  Convolutional Encoder/1 -> Rectangular QAM Modulator Baseband2/1, Display/1  "Before QAM"
  OFDM Modulator1/1 -> Modulated/1  "Sent"
  Pilot/1 -> OFDM Modulator1/2
  Rectangular QAM Modulator Baseband2/1 -> Vector Concatenate/1  "Before OFDM"

== system V2X_Core_Simulink_model/Subsystem/1//2 QPSK ==
  Bits : Inport
  Pilot : Inport  Port=2
  Constant2 : Constant  Commented=on  Value=[zeros(695,1)]  VectorParams1D=off  SampleTime=-1
  Convolutional Encoder : commcnvcod2/Convolutional Encoder  trellis=poly2trellis(7, [171 133])  opMode=Truncated (reset every frame)  DelayedResetAction=on  hasIniStPort=off  hasFinStPort=off  usePuncVector=on  punctureVector=[1;1]  reset=Unused parameter value
      settings: LibrarySourceBlock=|
      | commhdlcnvcod/Convolutional
      | Encoder
  Gain : Gain  Gain=1/sqrt(10)
  Matrix Concatenate : Concatenate  NumInputs=6  Mode=Multidimensional array  ConcatenateDimension=2
  OFDM Modulator1 : commofdm/OFDM Modulator  StatePerturbationForJacobian=1.0e-05  FFTLength=64  NumGuardBandCarriers=[6;5]  InsertDCNull=on  PilotInputPort=on  PilotCarrierIndices=[12; 26; 40; 54]  CyclicPrefixLength=16  Windowing=off  WindowLength=16  OversamplingFactor=1  NumSymbols=6  NumTransmitAntennas=1  SimulateUsing=Interpreted execution
  QPSK Modulator Baseband : commdigbbndpm3/QPSK Modulator Baseband  InType=Bit  Enc=Gray  Ph=pi/4  outDtype=double  outWordLen=16  outUDDataType=sfix(16)  outFracLenMode=Best precision  outFracLen=15  outDataTypeStr=double  outLastDataTypeStr=double
      settings: LibrarySourceBlock=|
      | commhdldigbbndpm/QPSK
      | Modulator
      | Baseband
  Random Interleaver : commblkintrlv2/Random Interleaver  StatePerturbationForJacobian=1.0e-05  N=576  seed=12345
  Reshape : Reshape  OutputDimensionality=Customize  OutputDimensions=[48,6]
  Vector Concatenate : Concatenate  Commented=on
  Modulated : Outport
  wires:
  OFDM Modulator1/1 -> Modulated/1  "OFDM modulated"
  QPSK Modulator Baseband/1 -> Gain/1
  Bits/1 -> Convolutional Encoder/1
  Convolutional Encoder/1 -> Random Interleaver/1
  Gain/1 -> Reshape/1  "After QAM Mod"
  Pilot/1 -> Matrix Concatenate/1, Matrix Concatenate/2, Matrix Concatenate/3, Matrix Concatenate/6, Matrix Concatenate/5, Matrix Concatenate/4
  Random Interleaver/1 -> QPSK Modulator Baseband/1
  Reshape/1 -> OFDM Modulator1/1
  Constant2/1 -> Vector Concatenate/2
  Matrix Concatenate/1 -> OFDM Modulator1/2

== system V2X_Core_Simulink_model/Subsystem/3//4 64 QAM ==
  Bits : Inport
  Pilot : Inport  Port=2
  Constant2 : Constant  Value=[zeros(32,1)']  VectorParams1D=off  SampleTime=-1
  Convolutional Encoder : commcnvcod2/Convolutional Encoder  trellis=poly2trellis(7, [171 133])  opMode=Truncated (reset every frame)  DelayedResetAction=on  hasIniStPort=off  hasFinStPort=off  usePuncVector=on  punctureVector=[1;1;0;1;1;0]  reset=Unused parameter value
      settings: LibrarySourceBlock=|
      | commhdlcnvcod/Convolutional
      | Encoder
  Display : Display
  Matrix Concatenate : Concatenate  Mode=Multidimensional array  ConcatenateDimension=2
  OFDM Modulator1 : commofdm/OFDM Modulator  StatePerturbationForJacobian=1.0e-05  FFTLength=64  NumGuardBandCarriers=[6;5]  InsertDCNull=on  PilotInputPort=on  PilotCarrierIndices=[12; 26; 40; 54]  CyclicPrefixLength=16  Windowing=off  WindowLength=16  OversamplingFactor=1  NumSymbols=2  NumTransmitAntennas=1  SimulateUsing=Interpreted execution
  Random Interleaver : commblkintrlv2/Random Interleaver  StatePerturbationForJacobian=1.0e-05  N=384  seed=12345
  Rectangular QAM Modulator Baseband2 : commdigbbndam3/Rectangular QAM Modulator Baseband  M=2^6  InType=Bit  Enc=Gray  Mapping=[0:15]  PowType=Average Power  MinDist=2  AvgPow=0.1  PeakPow=1  Ph=0  outDtype=double  outWordLen=16  outUDDataType=sfix(16)  outFracLenMode=Best precision  outFracLen=15  outDataTypeStr=double  outLastDataTypeStr=double
      settings: LibrarySourceBlock=|
      | commhdldigbbndam/Rectangular QAM
      | Modulator
      | Baseband
  Reshape : Reshape  OutputDimensionality=Customize  OutputDimensions=[48,2]
  Vector Concatenate : Concatenate
  Modulated : Outport
  wires:
  Rectangular QAM Modulator Baseband2/1 -> Vector Concatenate/1  "Before OFDM"
  OFDM Modulator1/1 -> Modulated/1  "Sent"
  Convolutional Encoder/1 -> Random Interleaver/1  "Before QAM"
  Constant2/1 -> Vector Concatenate/2
  Vector Concatenate/1 -> Reshape/1  "After QAM Mod"
  Bits/1 -> Convolutional Encoder/1  "Raw"
  Random Interleaver/1 -> Display/1, Rectangular QAM Modulator Baseband2/1
  Reshape/1 -> OFDM Modulator1/1
  Pilot/1 -> Matrix Concatenate/1, Matrix Concatenate/2
  Matrix Concatenate/1 -> OFDM Modulator1/2

== system V2X_Core_Simulink_model/Subsystem3/1//2 64 QAM1 ==
  Output : Inport
  Bit to Integer Converter2 : simulink/Logic and Bit Operations/Bit to Integer Converter  nbits=16  bitOrder=MSB first  signedOutputValues=Signed  outDtype=int16  outDtypeSigned=int16
  Complex to Real-Imag : ComplexToRealImag
  Display : Display
  Display2 : Display
  OFDM Demodulator : commofdm/OFDM Demodulator  StatePerturbationForJacobian=1.0e-05  FFTLength=1024  NumGuardBandCarriers=[0; 0]  RemoveDCCarrier=on  PilotOutputPort=on  PilotCarrierIndices=pilotInd  CyclicPrefixLength=512  OversamplingFactor=1  NumSymbols=1  NumReceiveAntennas=1  SimulateUsing=Interpreted execution
  Rectangular QAM Demodulator Baseband2 : commdigbbndam3/Rectangular QAM Demodulator Baseband  M=64  OutType=Bit  DecType=Hard decision  VarSource=Dialog  Variance=1  Dec=Gray  Mapping=[0:15]  PowType=Average Power  MinDist=2  AvgPow=42  PeakPow=1  Ph=0  outDtype1=int16  outDtype2=int16  derotateFactorWordLen=16  derotateFactorDataTypeStr=Inherit: Same word length as input  derotateFactorLastDataTypeStr=Inherit: Same word length as input  denormFactorWordLen=16  denormFactorDataTypeStr=Inherit: Same word length as input  denormFactorLastDataTypeStr=Inherit: Same word length as input  prodOutWordLen=32  prodOutOverflowMode=Wrap  prodOutRoundingMode=Floor  prodOutOvFlMode=off  prodOutOvFlModeLastStrValue=off  sumWordLen=32
      settings: LibrarySourceBlock=|
      | commhdldigbbndam/Rectangular QAM
      | Demodulator
      | Baseband
  Selector : Selector  InputPortWidth=983  IndexOptions=Index vector (dialog)  Indices=[1:96]  OutputSizes=1
  Selector1 : Selector  Commented=on  InputPortWidth=18  IndexOptions=Index vector (dialog)  Indices=[7:18]  OutputSizes=1
  Selector2 : Selector  Commented=on  InputPortWidth=18  IndexOptions=Index vector (dialog)  Indices=[1:6]  OutputSizes=1
  Vector Concatenate : Concatenate  Commented=on
  Viterbi Decoder : commcnvcod2/Viterbi Decoder  trellis=poly2trellis(7, [171 133])  isPunctured=off  punctureVector=[1;1;0;1;1;0;1;1;0;1;0;1;1;0;1;1;0;1]  erasures=off  dectype=Hard decision  nsdecb=4  runSigValErrCheck=off  tbdepth=96  opmode=Truncated  reset=off  delayedResetAction=on  smWordLength=16  outDataType=int16
      settings: LibrarySourceBlock=commhdlcnvcod/Viterbi Decoder
  Modulated : Outport
  wires:
  Selector2/1 -> Vector Concatenate/2
  Selector1/1 -> Vector Concatenate/1
  Bit to Integer Converter2/1 -> Modulated/1, Display2/1
  Complex to Real-Imag/1 -> Display/1
  Rectangular QAM Demodulator Baseband2/1 -> Viterbi Decoder/1  "After QAM"
  OFDM Demodulator/1 -> Selector/1  "After OFDM"
  Viterbi Decoder/1 -> Bit to Integer Converter2/1  "Raw"
  Selector/1 -> Rectangular QAM Demodulator Baseband2/1  "After OFDM"
  Output/1 -> OFDM Demodulator/1  "Sent"
  OFDM Demodulator/2 -> Complex to Real-Imag/1

== system V2X_Core_Simulink_model/Subsystem3/1//2 QPSK ==
  Output : Inport
  Bit to Integer Converter2 : simulink/Logic and Bit Operations/Bit to Integer Converter  nbits=16  bitOrder=MSB first  signedOutputValues=Signed  outDtype=int16  outDtypeSigned=int16
  Display : Display
  OFDM Demodulator1 : commofdm/OFDM Demodulator  Commented=on  StatePerturbationForJacobian=1.0e-05  FFTLength=64  NumGuardBandCarriers=[0; 0]  RemoveDCCarrier=on  PilotOutputPort=on  PilotCarrierIndices=[12; 26; 40; 54]  CyclicPrefixLength=32  OversamplingFactor=3  NumSymbols=1  NumReceiveAntennas=1  SimulateUsing=Interpreted execution
  OFDM Demodulator2 : commofdm/OFDM Demodulator  StatePerturbationForJacobian=1.0e-05  FFTLength=64  NumGuardBandCarriers=[6; 5]  RemoveDCCarrier=on  PilotOutputPort=on  PilotCarrierIndices=[12; 26; 40; 54]  CyclicPrefixLength=16  OversamplingFactor=1  NumSymbols=6  NumReceiveAntennas=1  SimulateUsing=Interpreted execution
  QPSK Demodulator Baseband : commdigbbndpm3/QPSK Demodulator Baseband  OutType=Bit  DecType=Hard decision  VarSource=Dialog  Variance=1  Dec=Gray  Ph=pi/4  outDtype1=Inherit via internal rule  outDtype2=Inherit via internal rule  derotateFactorWordLen=16  derotateFactorDataTypeStr=Inherit: Same word length as input  derotateFactorLastDataTypeStr=Inherit: Same word length as input
      settings: LibrarySourceBlock=|
      | commhdldigbbndpm/QPSK
      | Demodulator
      | Baseband
  Random Deinterleaver : commblkintrlv2/Random Deinterleaver  StatePerturbationForJacobian=1.0e-05  N=576  seed=12345
  Reshape : Reshape
  Selector : Selector  InputPortWidth=288  IndexOptions=Index vector (dialog)  Indices=[1:288]  OutputSizes=1
  Viterbi Decoder : commcnvcod2/Viterbi Decoder  trellis=poly2trellis(7, [171 133])  isPunctured=on  punctureVector=[1; 1]  erasures=off  dectype=Hard decision  nsdecb=4  runSigValErrCheck=off  tbdepth=30  opmode=Truncated  reset=off  delayedResetAction=on  smWordLength=16  outDataType=Smallest unsigned integer
      settings: LibrarySourceBlock=commhdlcnvcod/Viterbi Decoder
  Modulated : Outport
  wires:
  OFDM Demodulator2/2 -> Display/1
  OFDM Demodulator2/1 -> Reshape/1  "Before QAM Demod"
  Output/1 -> OFDM Demodulator2/1
  QPSK Demodulator Baseband/1 -> Random Deinterleaver/1
  Selector/1 -> QPSK Demodulator Baseband/1
  Bit to Integer Converter2/1 -> Modulated/1
  Viterbi Decoder/1 -> Bit to Integer Converter2/1
  Reshape/1 -> Selector/1
  Random Deinterleaver/1 -> Viterbi Decoder/1

== system V2X_Core_Simulink_model/Subsystem3/3//4 64 QAM ==
  Output : Inport
  Bit to Integer Converter2 : simulink/Logic and Bit Operations/Bit to Integer Converter  nbits=16  bitOrder=MSB first  signedOutputValues=Signed  outDtype=int16  outDtypeSigned=int16
  Complex to Real-Imag : ComplexToRealImag
  Display : Display
  Display1 : Display
  Display2 : Display
  OFDM Demodulator : commofdm/OFDM Demodulator  StatePerturbationForJacobian=1.0e-05  FFTLength=64  NumGuardBandCarriers=[6; 5]  RemoveDCCarrier=on  PilotOutputPort=on  PilotCarrierIndices=[12; 26; 40; 54]  CyclicPrefixLength=16  OversamplingFactor=1  NumSymbols=2  NumReceiveAntennas=1  SimulateUsing=Interpreted execution
  Random Deinterleaver : commblkintrlv2/Random Deinterleaver  StatePerturbationForJacobian=1.0e-05  N=384  seed=12345
  Rectangular QAM Demodulator Baseband2 : commdigbbndam3/Rectangular QAM Demodulator Baseband  M=64  OutType=Bit  DecType=Hard decision  VarSource=Dialog  Variance=1  Dec=Gray  Mapping=[0:15]  PowType=Average Power  MinDist=2  AvgPow=0.1  PeakPow=1  Ph=0  outDtype1=int16  outDtype2=int16  derotateFactorWordLen=16  derotateFactorDataTypeStr=Inherit: Same word length as input  derotateFactorLastDataTypeStr=Inherit: Same word length as input  denormFactorWordLen=16  denormFactorDataTypeStr=Inherit: Same word length as input  denormFactorLastDataTypeStr=Inherit: Same word length as input  prodOutWordLen=32  prodOutOverflowMode=Wrap  prodOutRoundingMode=Floor  prodOutOvFlMode=off  prodOutOvFlModeLastStrValue=off  sumWordLen=32
      settings: LibrarySourceBlock=|
      | commhdldigbbndam/Rectangular QAM
      | Demodulator
      | Baseband
  Reshape : Reshape
  Selector : Selector  InputPortWidth=96  IndexOptions=Index vector (dialog)  Indices=[1:64]  OutputSizes=1
  Selector1 : Selector  Commented=on  InputPortWidth=18  IndexOptions=Index vector (dialog)  Indices=[7:18]  OutputSizes=1
  Selector2 : Selector  Commented=on  InputPortWidth=18  IndexOptions=Index vector (dialog)  Indices=[1:6]  OutputSizes=1
  Vector Concatenate : Concatenate  Commented=on
  Viterbi Decoder : commcnvcod2/Viterbi Decoder  trellis=poly2trellis(7, [171 133])  isPunctured=on  punctureVector=[1;1;0;1;1;0]  erasures=off  dectype=Hard decision  nsdecb=4  runSigValErrCheck=off  tbdepth=60  opmode=Truncated  reset=off  delayedResetAction=on  smWordLength=16  outDataType=int16
      settings: LibrarySourceBlock=commhdlcnvcod/Viterbi Decoder
  Modulated : Outport
  wires:
  OFDM Demodulator/2 -> Complex to Real-Imag/1
  Output/1 -> OFDM Demodulator/1  "Sent"
  Selector/1 -> Rectangular QAM Demodulator Baseband2/1  "After OFDM"
  Viterbi Decoder/1 -> Bit to Integer Converter2/1  "Raw"
  OFDM Demodulator/1 -> Reshape/1  "After OFDM"
  Rectangular QAM Demodulator Baseband2/1 -> Random Deinterleaver/1  "After QAM"
  Complex to Real-Imag/1 -> Display/1
  Bit to Integer Converter2/1 -> Display2/1, Modulated/1
  Selector1/1 -> Vector Concatenate/1
  Selector2/1 -> Vector Concatenate/2
  Reshape/1 -> Selector/1
  Random Deinterleaver/1 -> Viterbi Decoder/1
  Complex to Real-Imag/2 -> Display1/1

== system V2X_Core_Simulink_model/Subsystem3/If Action Subsystem ==
  In1 : Inport
  Action Port : ActionPort  ActionPortLabel=case [ 1 ]:
  Actor1 : Outport
  wires:
  In1/1 -> Actor1/1

== system V2X_Core_Simulink_model/Subsystem3/If Action Subsystem1 ==
  In1 : Inport
  Action Port : ActionPort  ActionPortLabel=case [ 2 ]:
  Out1 : Outport
  wires:
  In1/1 -> Out1/1

== system V2X_Core_Simulink_model/Subsystem3/If Action Subsystem2 ==
  Actors : Inport
  Action Port : ActionPort  ActionPortLabel=case [ 3 ]:
  Out1 : Outport
  wires:
  Actors/1 -> Out1/1

== system V2X_Core_Simulink_model/Subsystem3/If Action Subsystem3 ==
  Actors : Inport
  Action Port : ActionPort  ActionPortLabel=case [ 4 ]:
  Out1 : Outport
  wires:
  Actors/1 -> Out1/1

== system V2X_Core_Simulink_model/Subsystem3/If Action Subsystem4 ==
  Actors : Inport
  Action Port : ActionPort  ActionPortLabel=case [ 5 ]:
  Out1 : Outport
  wires:
  Actors/1 -> Out1/1

== system V2X_Core_Simulink_model/Subsystem3/If Action Subsystem5 ==
  Actors : Inport
  Action Port : ActionPort  ActionPortLabel=case [ 6 ]:
  Out1 : Outport
  wires:
  Actors/1 -> Out1/1

== system V2X_Core_Simulink_model/Subsystem4/1//2 QPSK ==
  Bits : Inport
  Pilot : Inport  Port=2
  Constant : Constant  Value=zeros(3,1)
  OFDM Modulator1 : commofdm/OFDM Modulator  StatePerturbationForJacobian=1.0e-05  FFTLength=128  NumGuardBandCarriers=[0;0]  InsertDCNull=on  PilotInputPort=on  PilotCarrierIndices=[24; 52; 80; 108]  CyclicPrefixLength=32  Windowing=off  WindowLength=16  OversamplingFactor=3  NumSymbols=1  NumTransmitAntennas=1  SimulateUsing=Interpreted execution
  QPSK Modulator Baseband : commdigbbndpm3/QPSK Modulator Baseband  InType=Bit  Enc=Gray  Ph=pi/4  outDtype=double  outWordLen=16  outUDDataType=sfix(16)  outFracLenMode=Best precision  outFracLen=15  outDataTypeStr=double  outLastDataTypeStr=double
      settings: LibrarySourceBlock=|
      | commhdldigbbndpm/QPSK
      | Modulator
      | Baseband
  Vector Concatenate : Concatenate
  Modulated : Outport
  wires:
  Constant/1 -> Vector Concatenate/2
  Vector Concatenate/1 -> OFDM Modulator1/1
  Bits/1 -> QPSK Modulator Baseband/1
  QPSK Modulator Baseband/1 -> Vector Concatenate/1
  Pilot/1 -> OFDM Modulator1/2
  OFDM Modulator1/1 -> Modulated/1  "OFDM modulated"

== system V2X_Core_Simulink_model/Subsystem4/64 QAM ==
  Bits : Inport
  Pilot : Inport  Port=2
  Constant2 : Constant  Value=[zeros(59,1)']  SampleTime=-1
  Convolutional Encoder : commcnvcod2/Convolutional Encoder  trellis=poly2trellis(7, [171 133])  opMode=Continuous  DelayedResetAction=on  hasIniStPort=off  hasFinStPort=off  usePuncVector=on  punctureVector=puncture_vector  reset=Unused parameter value
      settings: LibrarySourceBlock=|
      | commhdlcnvcod/Convolutional
      | Encoder
  OFDM Modulator1 : commofdm/OFDM Modulator  StatePerturbationForJacobian=1.0e-05  FFTLength=128  NumGuardBandCarriers=[0;0]  InsertDCNull=on  PilotInputPort=on  PilotCarrierIndices=[24; 52; 80; 108]  CyclicPrefixLength=32  Windowing=off  WindowLength=16  OversamplingFactor=1  NumSymbols=1  NumTransmitAntennas=1  SimulateUsing=Interpreted execution
  Rectangular QAM Modulator Baseband2 : commdigbbndam3/Rectangular QAM Modulator Baseband  M=2^6  InType=Bit  Enc=Gray  Mapping=[0:15]  PowType=Average Power  MinDist=2  AvgPow=42  PeakPow=1  Ph=0  outDtype=double  outWordLen=16  outUDDataType=sfix(16)  outFracLenMode=Best precision  outFracLen=15  outDataTypeStr=double  outLastDataTypeStr=double
      settings: LibrarySourceBlock=|
      | commhdldigbbndam/Rectangular QAM
      | Modulator
      | Baseband
  Vector Concatenate : Concatenate
  Modulated : Outport
  wires:
  Vector Concatenate/1 -> OFDM Modulator1/1  "After QAM Mod"
  Constant2/1 -> Vector Concatenate/2
  Convolutional Encoder/1 -> Rectangular QAM Modulator Baseband2/1
  OFDM Modulator1/1 -> Modulated/1  "OFDM modulated"
  Bits/1 -> Convolutional Encoder/1
  Pilot/1 -> OFDM Modulator1/2
  Rectangular QAM Modulator Baseband2/1 -> Vector Concatenate/1  "After QAM Mod"
